simulink model "Problem4"  (R2020b)
settings: Solver=VariableStepAuto  StartTime=0.0  StopTime=10.0  RelTol=1e-3
settings Model: Creator=Sourav Kumar  LastModifiedBy=Sourav Kumar

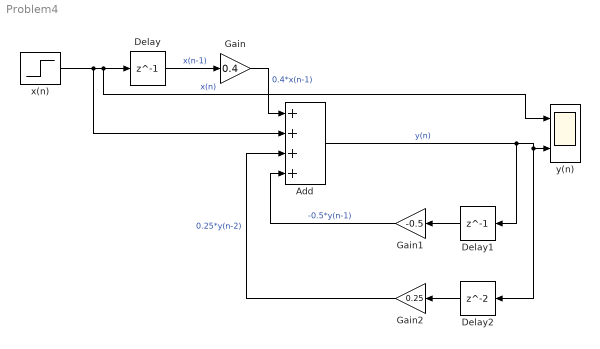
== system Problem4 ==
  Add : Sum  Inputs=++++
  Delay : Delay  DelayLength=1
  Delay1 : Delay  DelayLength=1
  Delay2 : Delay
  Gain : Gain  Gain=0.4
  Gain1 : Gain  Gain=-0.5
  Gain2 : Gain  Gain=0.25
  x(n) : Step  SampleTime=0
  y(n) : Scope  NumInputPorts=2
  wires:
  Add/1 -> Delay2/1, y(n)/2, Delay1/1  "y(n)"
  Gain/1 -> Add/1  "0.4*x(n-1)"
  Delay/1 -> Gain/1  "x(n-1)"
  Delay2/1 -> Gain2/1
  Gain1/1 -> Add/4  "-0.5*y(n-1)"
  x(n)/1 -> Add/2, y(n)/1, Delay/1  "x(n)"
  Gain2/1 -> Add/3  "0.25*y(n-2)"
  Delay1/1 -> Gain1/1
